simulink model "multi_stage_safety_aware"  (R2020b)
settings: Solver=FixedStepAuto  StartTime=0.0  StopTime=25  FixedStep=T_R  RelTol=1e-3
values from neighbouring files (symbols this model uses):
  a_max = F_max / m_R    (= 10)    [multi_stage_safety_aware_setup.m]    (also in stage_II_subsystem.m = 3)
  b0 = 20    [FSM.m]    (also in multi_stage_safety_aware_setup.m = 2 * sqrt(m_R * k0))
  E_max = 100    [multi_stage_safety_aware_setup.m]
  E_SAFE = 1    [multi_stage_safety_aware_setup.m]
  is_some_noise = false    [multi_stage_safety_aware_setup.m]
  j_max = 300    [multi_stage_safety_aware_setup.m]    (also in stage_II_subsystem.m = 30)
  k0 = 100    [FSM.m]    (also in multi_stage_safety_aware_setup.m)
  km = 100    [multi_stage_safety_aware_setup.m]
  m_R = 1    [multi_stage_safety_aware_setup.m]    (also in stage_II_subsystem.m)
  P_max = 100    [multi_stage_safety_aware_setup.m]
  P_SAFE = 0.5    [multi_stage_safety_aware_setup.m]
  s0 = 5    [multi_stage_safety_aware_setup.m]
  t_init = 0    [FSM.m]    (also in multi_stage_safety_aware_setup.m)
  T_R = 0.001    [multi_stage_safety_aware_setup.m]    (also in stage_II_subsystem.m)
  x_O = 1.5    [multi_stage_safety_aware_setup.m]
  x_R = 0    [multi_stage_safety_aware_setup.m]
libraries: dspstat3 x1
settings Model: NumberOfSteps=100  Creator=kika  LastModifiedBy=kika

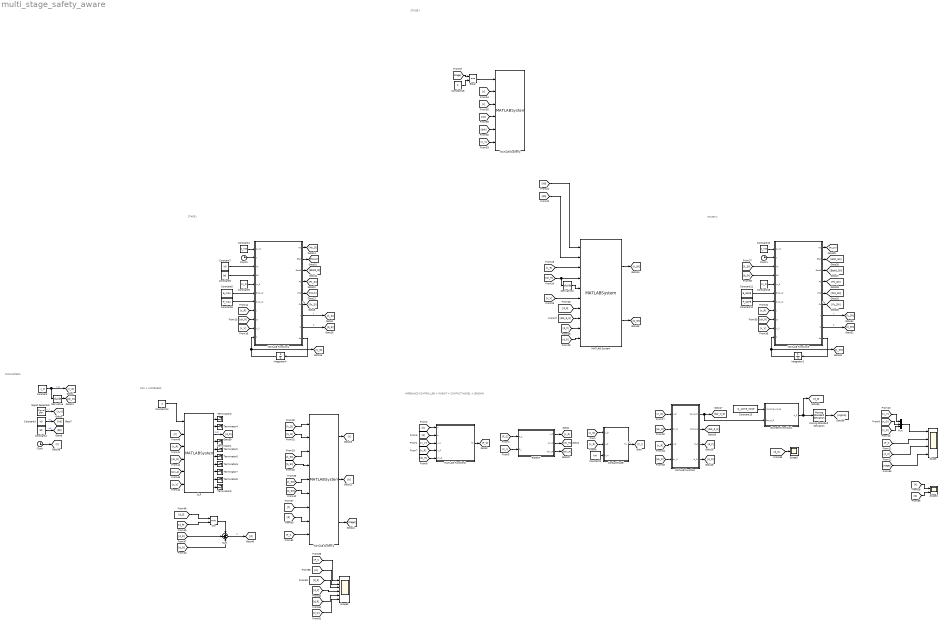
== system multi_stage_safety_aware ==
  note: PARAMETERS
  note: IMPEDANCE CONTROLLER + ROBOT + CONTACT MODEL + SENSING
  note: STAGE I
  note: STAGE II
  note: STAGE III
  note: FSM + HYSTERESIS
  Clock : Clock
  Clock1 : Clock
  Clock2 : Clock
  Constant : Constant  Value=x_O
  Constant1 : Constant  Value=t_init
  Constant10 : Constant  Value=t_init
  Constant11 : Constant  Value=E_SAFE
  Constant12 : Constant  Value=P_SAFE
  Constant13 : Constant  Value=is_some_noise
  Constant14 : Constant
  Constant15 : Constant  Value=m_R
  Constant16 : Constant  Value=2
  Constant2 : Constant  Value=km
  Constant3 : Constant  Value=k0
  Constant4 : Constant  Value=b0
  Constant5 : Constant  Value=E_max
  Constant6 : Constant  Value=P_max
  Constant7 : Constant  Value=k0
  Constant8 : Constant  Value=b0
  Constant9 : Constant  Value=m_R
  ContactModel : MATLAB Function  TreatAsAtomicUnit=on
  Derivative : Derivative
  Derivative1 : Derivative
  Equal : RelationalOperator  Operator===  OutDataTypeStr=boolean  RndMeth=Simplest
  Integrator1 : Integrator  InitialCondition=s0
  Integrator4 : Integrator  InitialCondition=s0
  MATLAB Function : MATLAB Function  TreatAsAtomicUnit=on
  MATLAB Function1 : MATLAB Function  TreatAsAtomicUnit=on
  MATLAB Function2 : MATLAB Function  TreatAsAtomicUnit=on
  MATLAB Function3 : MATLAB Function  TreatAsAtomicUnit=on
  MATLAB System : MATLABSystem  System=stage_II_subsystem  m_R=m_R  T_R=[T_R]  a_max=[a_max]  j_max=[j_max]  SimulateUsing=Code generation
      mask Type: stage_II_subsystem
      mask Display:
      | disp('stage_II_subsystem');
      | port_label('input',1,'k_SI');
      | port_label('input',2,'b_SI');
      | port_label('input',3,'x_R');
      | port_label('input',4,'dx_R');
      | port_label('input',5,'ddx_R');
      | port_label('input',6,'x_V');
      | port_label('input',7,'d_S');
      | port_label('input',8,'dot_d_S');
      | port_label('input',9,'d_P');
      | port_label('input',10,'d_O');
      | port_label('output',1,'k_SII');
      | port_label('output',2,'b_SII');
  MATLAB System1 : MATLABSystem  System=FSM  t_init=0  F_I_delta=0  d_delta=0  k0=k0  b0=b0  SimulateUsing=Code generation
      mask Type: FSM
      mask Display:
      | disp('FSM');
      | port_label('input',1,'k1');
      | port_label('input',2,'b1');
      | port_label('input',3,'k2');
      | port_label('input',4,'b2');
      | port_label('input',5,'k3');
      | port_label('input',6,'b3');
      | port_label('input',7,'t');
      | port_label('input',8,'d');
      | port_label('input',9,'F_I');
      | port_label('output',1,'k_');
      | port_label('output',2,'b_');
      | port_label('output',3,'stage');
  MATLAB System2 : MATLABSystem  System=braking_memory_trapezoid  a_max=a_max  j_max=j_max  T_R=T_R  x0_=x0  v0_=v0  k0=k0  b0=b0  SimulateUsing=Code generation
      mask Type: braking_memory_trapezoid
      mask Display:
      | disp('braking_memory_trapezoid');
      | port_label('input',1,'state');
      | port_label('input',2,'t');
      | port_label('input',3,'x');
      | port_label('input',4,'dx');
      | port_label('input',5,'ddx');
      | port_label('input',6,'x_V0');
      | port_label('output',1,'d_b0');
      | port_label('output',2,'d_b_j0');
      | port_label('output',3,'t_b0');
      | port_label('output',4,'h10');
      | port_label('output',5,'h20');
      | port_label('output',6,'h30');
      | port_label('output',7,'x0');
      | port_label('output',8,'v0');
      | port_label('output',9,'a0');
      | port_label('output',10,'t0');
  Min : MinMax  Inputs=2
  Moving Standard Deviation : dspstat3/Moving Standard Deviation  Method=Sliding window  ForgettingFactorPort=off  SpecifyWindowLength=on  WindowLength=l  ForgettingFactor=0.9  SimulateUsing=Code generation
      settings: SourceProductBaseCode=DS
  Mux : Mux  Inputs=3
  ROBOT : Subsystem
  Scope : Scope  NumInputPorts=4
  Scope1 : Scope  NumInputPorts=2
  Scope2 : Scope  NumInputPorts=6
  Scope3 : Scope
  Signal Generator : SignalGenerator  Amplitude=2  Units=rad/sec
  Sum : Sum  Inputs=+--
  Terminator{1..9} (9 alike) : Terminator
  d_R : MATLABSystem  System=braking_memory_rapid  a_max=a_max  j_max=j_max  T_R=T_R  x0_=x0  v0_=v0  k0=k0  b0=b0  SimulateUsing=Code generation
      mask Type: braking_memory_rapid
      mask Display:
      | disp('braking_memory_rapid');
      | port_label('input',1,'state');
      | port_label('input',2,'t');
      | port_label('input',3,'x');
      | port_label('input',4,'dx');
      | port_label('input',5,'ddx');
      | port_label('input',6,'x_V0');
      | port_label('output',1,'d_b0');
      | port_label('output',2,'d_b_j0');
      | port_label('output',3,'t_b0');
      | port_label('output',4,'h10');
      | port_label('output',5,'h20');
      | port_label('output',6,'h30');
      | port_label('output',7,'x0');
      | port_label('output',8,'v0');
      | port_label('output',9,'a0');
      | port_label('output',10,'t0');
  discrete time block : MATLAB Function  TreatAsAtomicUnit=on
  wires:
  Constant2/1 -> ContactModel/3(k_m)
  [x_O] -> ContactModel/1(x_O)
  [x_V] -> MATLAB Function2/3(x_V)
  [k] -> MATLAB Function2/1(k)
  [b] -> MATLAB Function2/2(b)
  ContactModel/1(F_I) -> [F_I]  "F_I"
  ROBOT/1(x_R) -> [x_R]
  ROBOT/2(dx_R) -> [dx_R]
  [F_C] -> ROBOT/1(F_C)
  [F_I] -> ROBOT/2(F_I)
  [x_R] -> ContactModel/2(x_R)
  MATLAB Function2/1(Fc) -> [F_C]
  [x_R] -> MATLAB Function2/4(x_R)
  [dx_R] -> MATLAB Function2/5(dx_R)
  Constant/1 -> Derivative/1, [x_O]  "x_O"
  Mux/1 -> Scope/1
  [x_O] -> Mux/2
  [x_R] -> Mux/3
  Signal Generator/1 -> [x_V]  "x_V"
  Constant4/1 -> [b0]  "b0"
  Constant3/1 -> [k0]  "k0"
  [F_I] -> Scope/2
  [F_C] -> Scope/3
  [x_V] -> Mux/1
  Constant7/1 -> MATLAB Function1/3(k0)
  MATLAB Function1/1(Hs) -> [Hs_SI]
  MATLAB Function1/7(k) -> [k_SI]  "k"
  MATLAB Function1/3(Etot0) -> [Etot0_SI]
  Constant8/1 -> MATLAB Function1/4(b0)
  Constant1/1 -> MATLAB Function1/1(t_init)
  MATLAB Function1/5(Pc0) -> [Pc0_SI]
  MATLAB Function1/4(Pc) -> [Pc_SI]
  Constant6/1 -> MATLAB Function1/7(Pmax0)
  MATLAB Function1/9(ds) -> Integrator4/1
  [dx_R] -> MATLAB Function1/9(dx)
  Constant5/1 -> MATLAB Function1/6(Emax0)
  [x_V] -> MATLAB Function1/10(x_V)
  Clock2/1 -> MATLAB Function1/2(t)
  Constant9/1 -> MATLAB Function1/5(m_R)
  [x_R] -> MATLAB Function1/8(x)
  Integrator4/1 -> MATLAB Function1/11(s), [s_SI]
  MATLAB Function1/2(Etot) -> [Etot_SI]
  MATLAB Function1/8(b) -> [b_SI]  "b"
  MATLAB Function1/6(Fc) -> [Fc_SI]  "Fc"
  [x_O] -> MATLAB Function/1(x_O)
  [x_R] -> MATLAB Function/3(x_R)
  MATLAB Function/1(bar_d_S) -> discrete time block/2(bar_d_S), [bar_d_S]
  MATLAB Function/4(d_O) -> [d_O]
  MATLAB Function/3(d_P) -> [d_P]
  MATLAB Function/2(dot_d_S) -> [dot_d_S]
  Derivative/1 -> [dx_O]
  MATLAB System1/1 -> [k]
  MATLAB System1/2 -> [b]
  MATLAB System/1 -> [k_SII]
  MATLAB System/2 -> [b_SII]
  [k0] -> MATLAB System/1
  [b0] -> MATLAB System/2
  [x_R] -> MATLAB System/3
  [dx_R] -> Derivative1/1, MATLAB System/4
  [x_V] -> MATLAB System/6
  [d_S] -> MATLAB System/7
  [dot_d_S] -> MATLAB System/8
  [d_P] -> MATLAB System/9
  [d_O] -> MATLAB System/10
  [dx_O] -> MATLAB Function/2(dx_O)
  MATLAB Function3/8(b) -> [b_SIII]  "b"
  Constant10/1 -> MATLAB Function3/1(t_init)
  MATLAB Function3/6(Fc) -> [Fc_SIII]  "Fc"
  Constant15/1 -> MATLAB Function3/5(m_R)
  MATLAB Function3/3(Etot0) -> [Etot0_SIII]
  MATLAB Function3/7(k) -> [k_SIII]  "k"
  Integrator1/1 -> MATLAB Function3/11(s), [s_SIII]
  Constant11/1 -> MATLAB Function3/6(Emax0)
  Constant12/1 -> MATLAB Function3/7(Pmax0)
  [dx_R] -> MATLAB Function3/9(dx)
  [x_V] -> MATLAB Function3/10(x_V)
  Clock1/1 -> MATLAB Function3/2(t)
  MATLAB Function3/4(Pc) -> [Pc_SIII]
  MATLAB Function3/2(Etot) -> [Etot_SIII]
  [x_R] -> MATLAB Function3/8(x)
  MATLAB Function3/9(ds) -> Integrator1/1
  MATLAB Function3/1(Hs) -> [Hs_SII]
  MATLAB Function3/5(Pc0) -> [Pc0_SIII]
  [b_SII] -> MATLAB Function3/4(b0)
  [k_SII] -> MATLAB Function3/3(k0)
  [dx_R] -> MATLAB Function/4(dx_R)
  Constant13/1 -> discrete time block/1(is_some_noise)
  discrete time block/1(d_S) -> [d_S], Moving Standard Deviation/1
  Moving Standard Deviation/1 -> [sigma]
  Derivative1/1 -> MATLAB System/5
  MATLAB System1/3 -> [stage]
  ROBOT/3(ddx_R) -> [ddx_R]
  Clock/1 -> [t]
  [t] -> MATLAB System2/2
  [ddx] -> MATLAB System2/5
  [x] -> MATLAB System2/3
  [x_V] -> MATLAB System2/6
  [dx] -> MATLAB System2/4
  [x_R] -> d_R/3
  Constant14/1 -> d_R/1
  [dx_R] -> d_R/4
  [ddx_R] -> d_R/5
  d_R/7 -> Terminator6/1
  [t] -> d_R/2
  d_R/1 -> Terminator3/1
  [x_V] -> d_R/6
  d_R/10 -> Terminator9/1
  d_R/3 -> [d_R]  "d_R"
  d_R/4 -> Terminator1/1
  d_R/6 -> Terminator5/1
  d_R/9 -> Terminator8/1
  d_R/8 -> Terminator7/1
  d_R/5 -> Terminator2/1
  d_R/2 -> Terminator4/1
  [d_P] -> Min/2
  Sum/1 -> [d]  "d"
  [d_S] -> Min/1
  [d_R] -> Sum/2
  [d_O] -> Sum/3
  Min/1 -> Sum/1
  [k_SII] -> MATLAB System1/3
  [b_SI] -> MATLAB System1/2
  [k_SI] -> MATLAB System1/1
  [b_SII] -> MATLAB System1/4
  [k_SIII] -> MATLAB System1/5
  [b_SIII] -> MATLAB System1/6
  [t] -> MATLAB System1/7
  [d] -> MATLAB System1/8
  [F_I] -> MATLAB System1/9
  [k] -> Scope1/1
  [b] -> Scope1/2
  [stage] -> Scope/4
  [d_P] -> Scope2/4
  [d_S] -> Scope2/3
  [d_R] -> Scope2/5
  [d] -> Scope2/2
  [d_O] -> Scope2/6
  [F_I] -> Scope2/1
  [d_S] -> Scope3/1
  [stage] -> Equal/1
  Constant16/1 -> Equal/2
  Equal/1 -> MATLAB System2/1

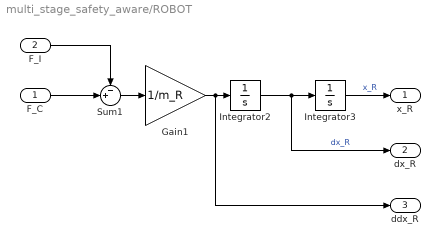
== system multi_stage_safety_aware/ROBOT ==
  F_C : Inport
  F_I : Inport  Port=2
  Gain1 : Gain  Gain=1/m_R
  Integrator2 : Integrator
  Integrator3 : Integrator  InitialCondition=x_R
  Sum1 : Sum  Inputs=-+|
  x_R : Outport
  dx_R : Outport  Port=2
  ddx_R : Outport  Port=3
  wires:
  Sum1/1 -> Gain1/1
  Gain1/1 -> ddx_R/1, Integrator2/1
  F_I/1 -> Sum1/1
  Integrator2/1 -> dx_R/1, Integrator3/1  "dx_R"
  Integrator3/1 -> x_R/1  "x_R"
  F_C/1 -> Sum1/2

== matlab function multi_stage_safety_aware/discrete time block ==
  settings: updateMethod=DISCRETE
  data: is_some_noise input; bar_d_S input; d_S output
function d_S = add_noise(is_some_noise, bar_d_S)
    
    d_S = bar_d_S;
    
    % generate some noise and add it to distance d_S
    % THINK ME: what about to add noise to dot_d_S?
    if is_some_noise
        noise   = 0 + randn(1) * 0.01;
        d_S = bar_d_S + noise;
    end

== matlab function multi_stage_safety_aware/ContactModel ==
  data: x_O input; x_R input; k_m input; F_I output
function F_I = ContactModel(x_O, x_R, k_m)

F_I = 0;
if x_R > x_O
    F_I = k_m * (x_R - x_O);
end

== matlab function multi_stage_safety_aware/MATLAB Function2 ==
  data: k input; b input; x_V input; Fc output; x_R input; dx_R input
function Fc = ImedanceController(k, b, x_V, x_R, dx_R)

Fc = k * (x_V - x_R) - b * dx_R;

== matlab function multi_stage_safety_aware/MATLAB Function1 ==
  data: t_init input; t input; k0 input; b0 input; m_R input; Hs output; Emax0 input; Pmax0 input; Etot output; Etot0 output; Pc output; Pc0 output; Fc output; x input; k output; b output; dx input; x_V input; s input; ds output
function [Hs, Etot, Etot0, Pc, Pc0, Fc, k, b, ds] = energy_aware_subsystem(t_init,t, k0, b0, m_R, Emax0, Pmax0, x, dx, x_V, s)
    %TODO `b` compute from critical damping 
    
    % initialisation time
    Emax = 1000;
    Pmax = 2000;
    if t > t_init
        Emax = Emax0;
        Pmax = Pmax0;
    end

    e = x_V - x;  % control error
    
    % Kinetic energy
    T = 0.5 * m_R * dx^2;

    % stiffness abjusting using initial Potential energy
    V0 = 0.5 * k0 * e^2;
    Etot0 = T + V0;
    k = k0;
    if Etot0 > Emax
        k = (Emax - T) / (0.5 * e^2);
    end

    % damping adjusting using new stiffness
    Fs = k * e;
    Fd0 = b0 * dx;
    Fc0 = Fs - Fd0;
    Pc0 = Fc0 * dx;
    b = b0;
    if Pc0 > Pmax
        b = (Fs * dx - Pmax) / dx^2;
    end

    % new control
    Fd = b * dx;
    Fc = Fs - Fd; % control without passivity

    % adjusted total Energy and Power
    V = 0.5 * k * e^2;
    Etot = T + V;
    Pc = Fc * dx;

    % Passivity
    eps = 0.1;
    Hs = 0.5 * s^2;

    u = -Fc * s / sqrt(2 * eps);    % or u = 0;
    if Hs >= eps || Pc < 0
        u = - Fc / s;
    end

    % total contol with passivity
    Fc = -u * s;
    ds = u * dx;

== matlab function multi_stage_safety_aware/MATLAB Function ==
  data: x_O input; dx_O input; bar_d_S output; dot_d_S output; d_P output; x_R input; d_O output; dx_R input
function [bar_d_S, dot_d_S, d_P, d_O] = sensor(x_O, dx_O, x_R, dx_R)

    bar_d_S = abs(x_R - x_O);
    dot_d_S = dx_R - dx_O;
    
    d_O = 0;
    d_P = 99;

== matlab function multi_stage_safety_aware/MATLAB Function3 ==
  data: t_init input; t input; k0 input; b0 input; m_R input; Hs output; Emax0 input; Pmax0 input; Etot output; Etot0 output; Pc output; Pc0 output; Fc output; x input; k output; b output; dx input; x_V input; s input; ds output
function [Hs, Etot, Etot0, Pc, Pc0, Fc, k, b, ds] = energy_aware_subsystem(t_init,t, k0, b0, m_R, Emax0, Pmax0, x, dx, x_V, s)
    
    % initialisation time
    Emax = 1000;
    Pmax = 2000;
    if t > t_init
        Emax = Emax0;
        Pmax = Pmax0;
    end

    e = x_V - x;  % control error
    
    % Kinetic energy
    T = 0.5 * m_R * dx^2;

    % stiffness abjusting using initial Potential energy
    V0 = 0.5 * k0 * e^2;
    Etot0 = T + V0;
    k = k0;
    if Etot0 > Emax
        k = (Emax - T) / (0.5 * e^2);
    end

    % damping adjusting using new stiffness
    Fs = k * e;
    Fd0 = b0 * dx;
    Fc0 = Fs - Fd0;
    Pc0 = Fc0 * dx;
    b = b0;
    if Pc0 > Pmax
        b = (Fs * dx - Pmax) / dx^2;
    end

    % new control
    Fd = b * dx;
    Fc = Fs - Fd; % control without passivity

    % adjusted total Energy and Power
    V = 0.5 * k * e^2;
    Etot = T + V;
    Pc = Fc * dx;

    % Passivity
    eps = 0.1;
    Hs = 0.5 * s^2;

    u = -Fc * s / sqrt(2 * eps);    % or u = 0;
    if Hs >= eps || Pc < 0
        u = - Fc / s;
    end

    % total contol with passivity
    Fc = -u * s;
    ds = u * dx;
